simulink model "Hybrid_Microgrid_EMS"  (R2026a)
settings: Solver=VariableStepAuto

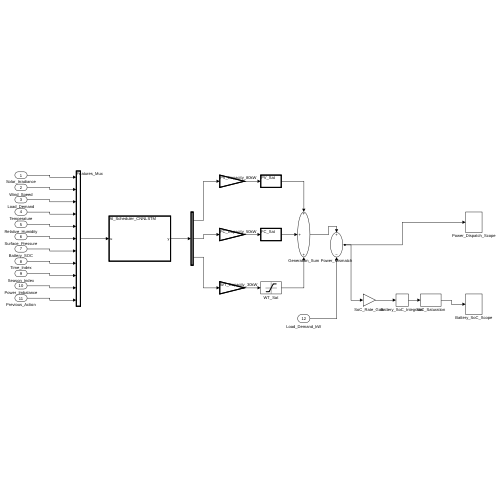
[thumbnail: Simulink's stored preview of the top-level diagram]
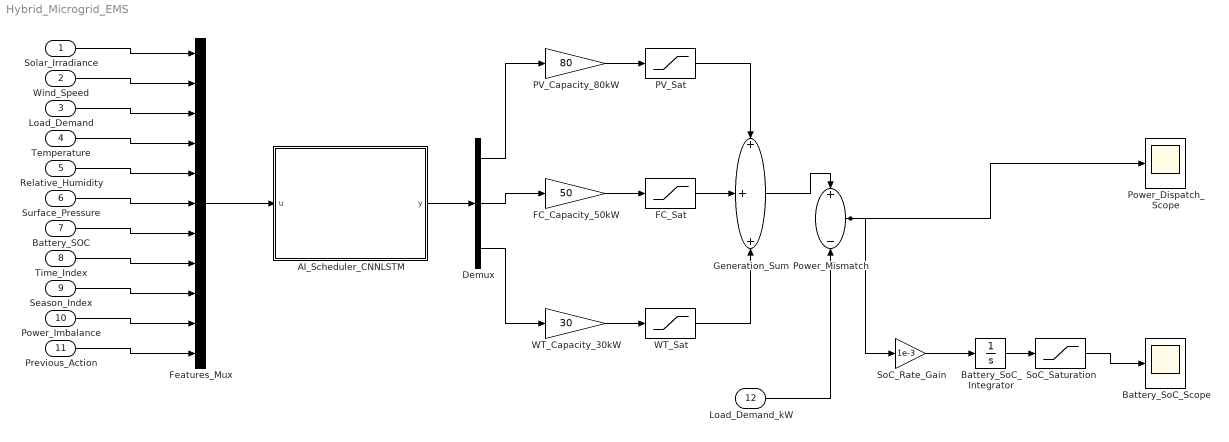
== system Hybrid_Microgrid_EMS ==
  Solar_Irradiance : Inport
  Wind_Speed : Inport  Port=2
  Load_Demand : Inport  Port=3
  Temperature : Inport  Port=4
  Relative_Humidity : Inport  Port=5
  Surface_Pressure : Inport  Port=6
  Battery_SOC : Inport  Port=7
  Time_Index : Inport  Port=8
  Season_Index : Inport  Port=9
  Power_Imbalance : Inport  Port=10
  Previous_Action : Inport  Port=11
  Load_Demand_kW : Inport  Port=12
  AI_Scheduler_CNNLSTM : MATLAB Function  TreatAsAtomicUnit=on
  Battery_SoC_Integrator : Integrator  InitialCondition=0.5
  Battery_SoC_Scope : Scope
  Demux : Demux  Outputs=3
  FC_Capacity_50kW : Gain  Gain=50
  FC_Sat : Saturate  UpperLimit=50  LowerLimit=0
  Features_Mux : Mux  Inputs=11
  Generation_Sum : Sum  Inputs=+++
  PV_Capacity_80kW : Gain  Gain=80
  PV_Sat : Saturate  UpperLimit=80  LowerLimit=0
  Power_Dispatch_Scope : Scope
  Power_Mismatch : Sum  Inputs=+-
  SoC_Rate_Gain : Gain  Gain=1e-3
  SoC_Saturation : Saturate  UpperLimit=0.9  LowerLimit=0.2
  WT_Capacity_30kW : Gain  Gain=30
  WT_Sat : Saturate  UpperLimit=30  LowerLimit=0
  wires:
  Solar_Irradiance/1 -> Features_Mux/1
  Wind_Speed/1 -> Features_Mux/2
  Load_Demand/1 -> Features_Mux/3
  Temperature/1 -> Features_Mux/4
  Relative_Humidity/1 -> Features_Mux/5
  Surface_Pressure/1 -> Features_Mux/6
  Battery_SOC/1 -> Features_Mux/7
  Time_Index/1 -> Features_Mux/8
  Season_Index/1 -> Features_Mux/9
  Power_Imbalance/1 -> Features_Mux/10
  Previous_Action/1 -> Features_Mux/11
  Features_Mux/1 -> AI_Scheduler_CNNLSTM/1(u)
  AI_Scheduler_CNNLSTM/1(y) -> Demux/1
  Demux/1 -> PV_Capacity_80kW/1
  Demux/2 -> FC_Capacity_50kW/1
  Demux/3 -> WT_Capacity_30kW/1
  PV_Capacity_80kW/1 -> PV_Sat/1
  FC_Capacity_50kW/1 -> FC_Sat/1
  WT_Capacity_30kW/1 -> WT_Sat/1
  PV_Sat/1 -> Generation_Sum/1
  FC_Sat/1 -> Generation_Sum/2
  WT_Sat/1 -> Generation_Sum/3
  Generation_Sum/1 -> Power_Mismatch/1
  Load_Demand_kW/1 -> Power_Mismatch/2
  Power_Mismatch/1 -> SoC_Rate_Gain/1, Power_Dispatch_Scope/1
  SoC_Rate_Gain/1 -> Battery_SoC_Integrator/1
  Battery_SoC_Integrator/1 -> SoC_Saturation/1
  SoC_Saturation/1 -> Battery_SoC_Scope/1

== matlab function Hybrid_Microgrid_EMS/AI_Scheduler_CNNLSTM ==
  data: u input; y output
function y = predictAI(u)
%#codegen
coder.extrinsic('predict','load');
persistent net
if isempty(net)
    s = load('Best_Microgrid_Scheduler.mat', 'bestNet');
    net = s.bestNet;
end
y = zeros(3,1);
y = predict(net, u);
end
